simulink model "twolink_inv_base"  (R2017b)
settings: Solver=VariableStepAuto  StartTime=0.0  StopTime=20  RelTol=1e-3
values from neighbouring files (symbols this model uses):
  h = diff(x)    [dfdx.m]    (also in inv_control.m = -m2*l1*lc2*sin(q2); twolink_ftraj.m = 0.1; twolink_valid.m = 0.1)
libraries: roblocks x1
settings Model: Creator=sathish  LastModifiedBy=sathish

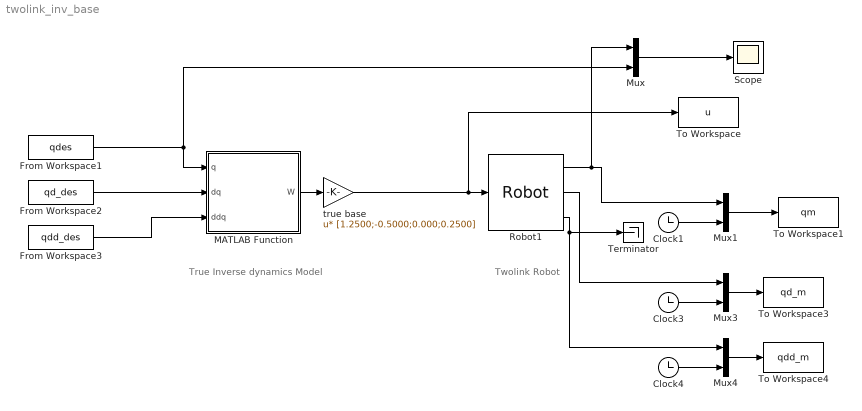
== system twolink_inv_base ==
  note: True Inverse dynamics Model
  note: Twolink Robot
  Clock1 : Clock
  Clock3 : Clock
  Clock4 : Clock
  From Workspace1 : FromWorkspace  VariableName=qdes  SampleTime=0
  From Workspace2 : FromWorkspace  VariableName=qd_des  SampleTime=0
  From Workspace3 : FromWorkspace  VariableName=qdd_des  SampleTime=0
  MATLAB Function : MATLAB Function  TreatAsAtomicUnit=on
  Mux{,1,3..4} (4 alike) : Mux  Inputs=2
  Robot1 : roblocks/Arm/Robot  robot=twolink_mod  q0=[0 0]
  Scope : Scope
  Terminator : Terminator
  To Workspace : ToWorkspace  VariableName=u  SampleTime=h
      settings: Save2DSignal=2-D array (concatenate along first dimension)
  To Workspace1 : ToWorkspace  VariableName=qm  SaveFormat=Timeseries  SampleTime=h
  To Workspace3 : ToWorkspace  VariableName=qd_m  SaveFormat=Timeseries  SampleTime=h
  To Workspace4 : ToWorkspace  VariableName=qdd_m  SaveFormat=Timeseries  SampleTime=h
  true base : Gain  Gain=[1.2500;-0.5000;0.000;0.2500]  Multiplication=Matrix(u*K)
  wires:
  Robot1/1 -> Mux1/1, Mux/1
  Clock4/1 -> Mux4/2
  Robot1/2 -> Mux3/1
  MATLAB Function/1(W) -> true base/1
  Clock3/1 -> Mux3/2
  Clock1/1 -> Mux1/2
  Mux3/1 -> To Workspace3/1
  From Workspace3/1 -> MATLAB Function/3(ddq)
  true base/1 -> To Workspace/1, Robot1/1
  Robot1/3 -> Mux4/1, Terminator/1
  Mux/1 -> Scope/1
  Mux4/1 -> To Workspace4/1
  From Workspace1/1 -> MATLAB Function/1(q), Mux/2
  From Workspace2/1 -> MATLAB Function/2(dq)
  Mux1/1 -> To Workspace1/1

== matlab function twolink_inv_base/MATLAB Function ==
  data: q input; W output; dq input; ddq input
function W = Regressor(q,dq,ddq)
x0 = ((dq(1))*(dq(1)));
x1 = ddq(1) + ddq(2);
x2 = sin(q(2));
x3 = dq(1)*x2;
x4 = dq(1) + dq(2);
x5 = cos(q(2));
x6 = ddq(1)*x5 - dq(2)*x3 + x3*x4;
x7 = -((x4)*(x4));
x8 = dq(1)*x5;
x9 = ddq(1)*x2 + dq(2)*x8;
x10 = x4*x8;
x11 = x10 - x9;
H = zeros(2,20);
  H(1) = 0;
  H(2) = 0;
  H(3) = 0;
  H(4) = 0;
  H(5) = 0;
  H(6) = ddq(1);
  H(7) = 2*ddq(1);
  H(8) = 0;
  H(8) = 0;
  H(10) = ddq(1);
  H(11) = 0;
  H(12) = 0;
  H(13) = 0;
  H(14) = 0;
  H(15) = 0;
  H(16) = x1;
  H(17) = x1*x5 + x2*x7 + x6;
  H(18) = -x1*x2 + x11 + x5*x7;
  H(19) = 0;
  H(20) = x2*(-x10 + x9) + x5*x6;
  H(21) = 0;
  H(22) = 0;
  H(23) = 0;
  H(24) = 0;
  H(25) = 0;
  H(26) = 0;
  H(27) = 0;
  H(28) = 0;
  H(29) = 0;
  H(30) = 0;
  H(31) = 0;
  H(32) = 0;
  H(33) = 0;
  H(34) = 0;
  H(35) = 0;
  H(36) = x1;
  H(37) = x6;
  H(38) = x11;
  H(39) = 0;
  H(40) = 0;
  Wl = zeros(2,20);
  k = 1;
     for i = 1:2
         for j = 1:20
             Wl(i,j) = H(k); 
             k = k+1;
         end
     end
     Wb1 = Wl(:,6);
     Wb2 = Wl(:,17);
     Wb3 = Wl(:,18);
     Wb4 = Wl(:,16);
     W = [Wb1,Wb2,Wb3,Wb4];
end
